simulink model "Our_SMC_Controller"  (R2019a)
settings: Solver=ode4  StartTime=0.0  StopTime=50  FixedStep=0.01  RelTol=1e-3
settings Model: Creator=Ashraf  LastModifiedBy=Ashraf
settings SolverCC: NumberNewtonIterations=2

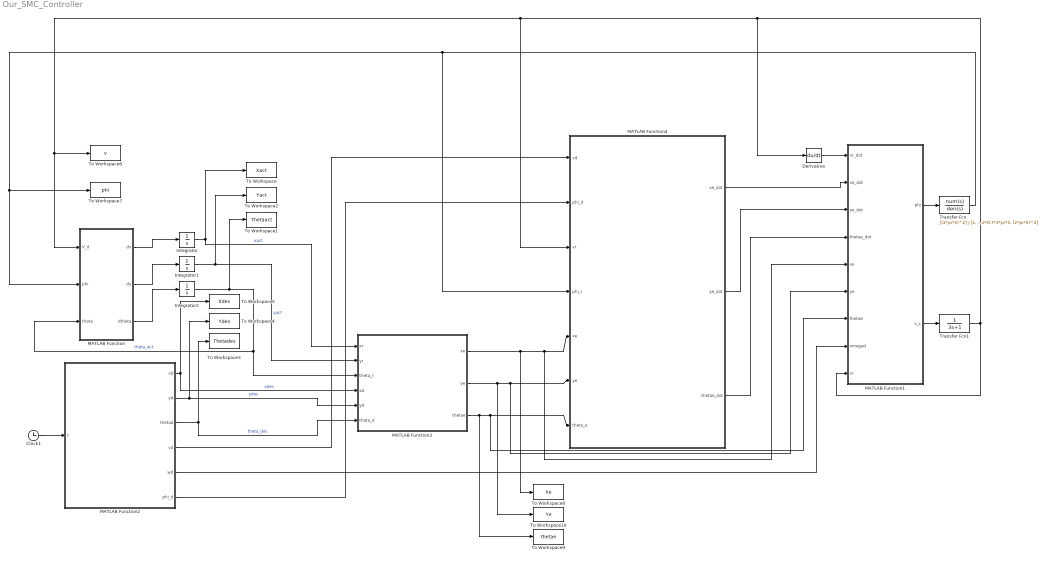
== system Our_SMC_Controller ==
  Clock1 : Clock
  Derivative : Derivative
  Integrator : Integrator  InitialCondition=2
  Integrator1 : Integrator
  Integrator2 : Integrator  InitialCondition=pi/2
  MATLAB Function : MATLAB Function  TreatAsAtomicUnit=on
  MATLAB Function1 : MATLAB Function  TreatAsAtomicUnit=on
  MATLAB Function2 : MATLAB Function  TreatAsAtomicUnit=on
  MATLAB Function3 : MATLAB Function  TreatAsAtomicUnit=on
  MATLAB Function4 : MATLAB Function  TreatAsAtomicUnit=on
  To Workspace : ToWorkspace  VariableName=Xact  SampleTime=-1
  To Workspace1 : ToWorkspace  VariableName=Thetaact  SampleTime=-1
  To Workspace10 : ToWorkspace  VariableName=Ye  SampleTime=-1
  To Workspace2 : ToWorkspace  VariableName=Yact  SampleTime=-1
  To Workspace3 : ToWorkspace  VariableName=Thetades  SampleTime=-1
  To Workspace4 : ToWorkspace  VariableName=Ydes  SampleTime=-1
  To Workspace5 : ToWorkspace  VariableName=Xdes  SampleTime=-1
  To Workspace6 : ToWorkspace  VariableName=v  SampleTime=-1
  To Workspace7 : ToWorkspace  VariableName=phi  SampleTime=-1
  To Workspace8 : ToWorkspace  VariableName=Xe  SampleTime=-1
  To Workspace9 : ToWorkspace  VariableName=thetae  SampleTime=-1
  Transfer Fcn : TransferFcn  Numerator=[(2*pi*5)^2]  Denominator=[1, 2*0.7*2*pi*5, (2*pi*5)^2]
  Transfer Fcn1 : TransferFcn  Denominator=[3, 1]  AbsoluteTolerance=10^-9
  wires:
  MATLAB Function/1(dx) -> Integrator/1
  MATLAB Function/2(dy) -> Integrator1/1
  MATLAB Function/3(dtheta) -> Integrator2/1
  Integrator/1 -> MATLAB Function3/1(xr), To Workspace/1  "xact"
  Integrator1/1 -> To Workspace2/1, MATLAB Function3/2(yr)  "yact"
  MATLAB Function2/1(xd) -> MATLAB Function3/4(xd), To Workspace5/1  "xdes"
  MATLAB Function2/2(yd) -> MATLAB Function3/5(yd), To Workspace4/1  "ydes"
  MATLAB Function2/3(thetad) -> MATLAB Function3/6(theta_d), To Workspace3/1  "theta_des"
  MATLAB Function3/1(xe) -> To Workspace8/1, MATLAB Function1/5(xe), MATLAB Function4/5(xe)
  MATLAB Function3/2(ye) -> To Workspace10/1, MATLAB Function1/6(ye), MATLAB Function4/6(ye)
  MATLAB Function3/3(thetae) -> To Workspace9/1, MATLAB Function1/7(thetae), MATLAB Function4/7(theta_e)
  MATLAB Function4/1(xe_dot) -> MATLAB Function1/2(xe_dot)
  MATLAB Function4/2(ye_dot) -> MATLAB Function1/3(ye_dot)
  MATLAB Function4/3(thetae_dot) -> MATLAB Function1/4(thetae_dot)
  MATLAB Function2/6(phi_d) -> MATLAB Function4/2(phi_d)
  MATLAB Function2/4(vd) -> MATLAB Function4/1(vd)
  MATLAB Function2/5(wd) -> MATLAB Function1/8(omegad)
  Clock1/1 -> MATLAB Function2/1(t)
  MATLAB Function1/1(phi) -> Transfer Fcn/1
  MATLAB Function1/2(v_c) -> Transfer Fcn1/1
  Integrator2/1 -> To Workspace1/1, MATLAB Function/3(theta), MATLAB Function3/3(theta_r)  "theta_act"
  Derivative/1 -> MATLAB Function1/1(vr_dot)
  Transfer Fcn/1 -> MATLAB Function4/4(phi_r), To Workspace7/1, MATLAB Function/2(phi)
  Transfer Fcn1/1 -> MATLAB Function1/9(vr), Derivative/1, To Workspace6/1, MATLAB Function/1(V_d), MATLAB Function4/3(vr)

== matlab function Our_SMC_Controller/MATLAB Function1 ==
  data: vr_dot input; phi output; xe_dot input; ye_dot input; thetae_dot input; xe input; v_c output; ye input; thetae input; omegad input; vr input
function [phi, v_c] = sliding_mode_control(vr_dot, xe_dot, ye_dot, thetae_dot, xe, ye, thetae, omegad, vr)
    % Initialize outputs to scalar dimensions for Simulink compatibility
    dv_c = 0.0000; % Scalar initialization
    phi = 0.000;  % Scalar initialization

    % Parameters definition
    L = 0.27;       % Wheelbase length
    domegad = 0;    % Desired angular velocity derivative
    vd_dot = 0;     % Desired velocity derivative

    % Gains
    k0 = 0.05;
    k1 = 0.25;
    k2 = 0.5;
    % Control parameters
    p1 = 1;
    p2 = 1;
    q1 = 1;
    q2 = 1;
    % Sliding surfaces
    s1 = xe_dot + k1 * xe;                      
    s2 = ye_dot + k2 * ye + k0 * sgn(ye) * thetae;  

    % Steering angle limit
    
    MAX_delta = pi/2.1;

        if abs(cos(thetae)) < 1e-3
        adjusted_cos = 1e-3; % Avoid zero and maintain consistent sign
        else
        adjusted_cos = cos(thetae);
        end

    % Control laws
    v_c = 1 / adjusted_cos * (-q1 * s1 - p1 * saturate(s1,-0.05,0.05) - k1 * xe_dot - domegad * ye ...
            - omegad * ye_dot + vr * thetae_dot * sin(thetae) + vd_dot);
    v_c = saturate(v_c, -0.3,0.3); % Example: Forward motion only, 0 to 2 m/s
    

    phi = atan((L / vr) * omegad + L / (vr * (vr * cos(thetae) + k0 * saturate(ye,-0.05,0.05))) ...
            * (-q2 * s2 - p2 * saturate(s2,-0.05,0.05) - k2 * ye_dot - vr_dot * sin(thetae) ...
            + domegad * xe + omegad * xe_dot));
    
    % Apply saturation to steering angle
    phi = saturate(phi, -MAX_delta, MAX_delta);    
end


% Saturation function
function [saturated_x] = saturate(x, lb, ub)
    % Ensures the value x stays within bounds [lb, ub]
    saturated_x = min(ub, max(lb, x));
end

function [ sgn ] = sgn( x )
%SGN %analytical sign approximation function
sgn=tanh(10*x);

end

== matlab function Our_SMC_Controller/MATLAB Function ==
  data: V_d input; dx output; phi input; theta input; dy output; dtheta output
function [dx, dy, dtheta] = kinematics(V_d, phi, theta)
    % Compute derivatives based on kinematic equations
    L = 0.27;
    
    dx = V_d * cos(theta);
    dy = V_d * sin(theta);
    dtheta = V_d / L * tan(phi);

end

== matlab function Our_SMC_Controller/MATLAB Function2 ==
  data: xd output; yd output; thetad output; vd output; wd output; phi_d output; t input
function [xd, yd, thetad, vd, wd, phi_d] = desiredTrajectory(t)
    % Parameters
    v_max = 0.3; % Maximum linear velocity (m/s)
    radius = 0.5; % Radius of the quarter-circle curve (m)
    L = 0.27;    % Vehicle wheelbase (m)
    horizontal_length = 4; % Length of the horizontal line (meters)
    vertical_length = 3;   % Length of the vertical line (meters)
    omega_curve = 0.2; % Angular velocity during the curve (rad/s)

    % Time intervals for each segment
    t_horizontal = horizontal_length / v_max; % Time for horizontal motion
    t_curve = pi / (2 * omega_curve);         % Time for quarter-circle curve
    t_vertical = vertical_length / v_max;    % Time for vertical motion

    % Total trajectory time
    t1 = t_horizontal; % End of horizontal motion
    t2 = t1 + t_curve; % End of quarter-circle curve
    t3 = t2 + t_vertical; % End of vertical motion

    % Initialize outputs
    xd = 0; yd = 0; thetad = 0;
    vd = v_max; wd = 0; phi_d = 0;

    % Determine current segment
    if t <= t1
        % Horizontal motion
        xd = v_max * t;
        yd = 0;
        thetad = 0; % Facing right
        vd = v_max; wd = 0;
        phi_d = 0;
    elseif t <= t2
        % Quarter-circle curve
        delta_t = t - t1;
        theta = omega_curve * delta_t; % Angle swept by the car
        xd = horizontal_length + radius * sin(theta);
        yd = radius * (1 - cos(theta));
        thetad = theta; % Orientation matches the curve
        vd = v_max; wd = omega_curve;
        phi_d = saturate(atan((L * wd) / vd), -pi / 2.1, pi / 2.1);
    elseif t <= t3
        % Vertical motion
        delta_t = t - t2;
        xd = horizontal_length + radius;
        yd = radius + v_max * delta_t;
        thetad = pi / 2; % Facing up
        vd = v_max; wd = 0;
        phi_d = 0;
    else
        % Stop at the end of the vertical line
        xd = horizontal_length + radius;
        yd = radius + vertical_length;
        thetad = pi / 2; % Facing up
        vd = 0; wd = 0;
        phi_d = 0;
    end
end

% Saturation function
function [saturated_x] = saturate(x, lb, ub)
    % Ensures the value x stays within bounds [lb, ub]
    saturated_x = min(ub, max(lb, x));
end

== matlab function Our_SMC_Controller/MATLAB Function3 ==
  data: xr input; xe output; yr input; theta_r input; xd input; yd input; theta_d input; ye output; thetae output
function [xe, ye, thetae] = calculateError(xr, yr, theta_r, xd, yd, theta_d)
    % Function to calculate the error in the local desired frame.
    %
    % Inputs:
    % xr, yr     - Robot's current position in the global frame.
    % theta_r    - Robot's current orientation in radians.
    % xd, yd     - Desired position in the global frame.
    % theta_d    - Desired orientation in radians.
    %
    % Outputs:
    % xe, ye     - Position errors in the desired frame.
    % theta_e    - Orientation error.
    
    % Calculate the relative errors in the global frame
    delta_x = xr - xd; % Difference in x
    delta_y = yr - yd; % Difference in y
    delta_theta = theta_r - theta_d; % Orientation error
    
    % Rotation matrix to transform global errors to the local desired frame
    Rot_desired = [cos(theta_d), sin(theta_d), 0; 
                  -sin(theta_d), cos(theta_d), 0; 
                   0,            0,           1];

    % Relative error vector in the global frame
    e_global = [delta_x; delta_y; delta_theta];
    
    % Transform the global errors to the local desired frame
    e_local = Rot_desired * e_global;

    % Extract the local errors
    xe = e_local(1);
    ye = e_local(2);
    thetae = e_local(3);
end

== matlab function Our_SMC_Controller/MATLAB Function4 ==
  data: vd input; phi_d input; xe_dot output; vr input; phi_r input; xe input; ye input; theta_e input; ye_dot output; thetae_dot output
function [xe_dot, ye_dot, thetae_dot] = calculate_error_derivative(vd, phi_d, vr, phi_r, xe, ye, theta_e)
    % Inputs:
    % vd       - Desired linear velocity
    % vr       - Reference linear velocity
    % xe, ye   - Position error in x and y
    % theta_e  - Heading angle error
    % phi_d    - Steering angle of the desired path
    % phi_r    - Steering angle of the reference path
    % l        - Wheelbase length of the vehicle

    % Outputs:
    % x_dot    - Derivative of x error
    % y_dot    - Derivative of y error
    % theta_dot - Derivative of theta error
    l = 0.27;
    % Compute x_dot
    xe_dot = -vd + vr * cos(theta_e) + ye * (vd / l) * tan(phi_d);
    %xe_dot = -vr + vd * cos(theta_e) + ye * (vr / l) * tan(phi_d);
    % Compute y_dot
     ye_dot = vr * sin(theta_e) - xe * (vd / l) * tan(phi_d);
    %ye_dot = vd * sin(theta_e) - xe * (vr / l) * tan(phi_d);
    % Compute theta_dot
    thetae_dot = (vr / l) * tan(phi_r) - xe * (vd / l) * tan(phi_d);
    %thetae_dot = (vd / l) * tan(phi_r) - xe * (vr / l) * tan(phi_d);
end
